simulink model "vel_loop_Bmat"  (Simulink 7.2)
settings: Solver=FixedStepDiscrete  StartTime=0.0  StopTime=0  FixedStep=MACH.dt  RelTol=1e-3
undefined symbols (not defined in the file or in its folder): att_trim_IC, MACH, MACH_mass_IC, MACH_vel_IC, obac_params, u_obac_IC, x_obac_IC
libraries: utility_lib x2, model_lib x2, models x1
settings Model: Creator=E183308  LastModifiedBy=E183308
settings DataIOCC: ExternalInput=[0 d_in]  LoadExternalInput=on  SignalLogging=off  SaveTime=off
settings OptimizationCC: InitFltsAndDblsToZero=on
settings DebuggingCC: SaveWithParameterizedLinksMsg=none  SignalResolutionControl=TryResolveAllWithWarning  InheritedTsInSrcMsg=none  MultiTaskDSMMsg=warning  MultiTaskCondExecSysMsg=none
settings RTWCC: IncludeERTFirstTime=on
settings GRTTargetCC: TargetFcnLib=ansi_tfl_tmw.mat

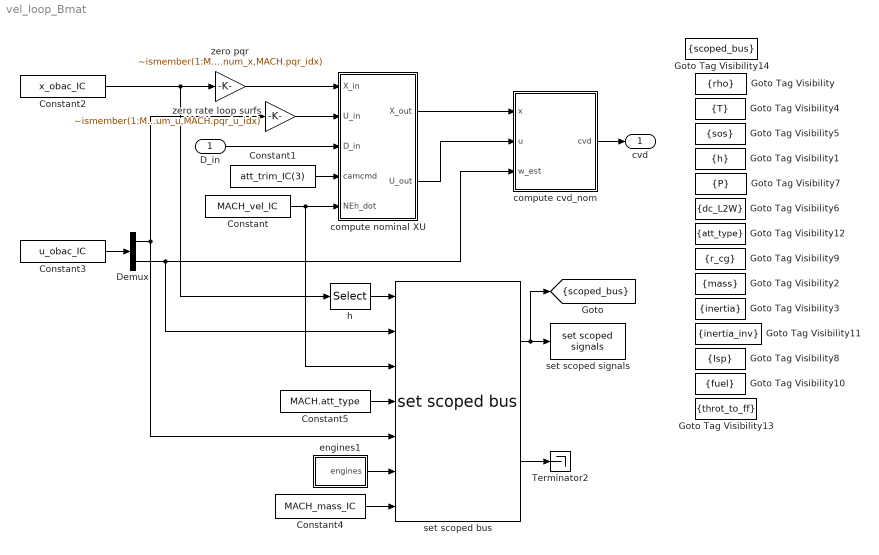
== system vel_loop_Bmat ==
  D_in : Inport  OutDataType=sfix(16)  OutScaling=2^0
  Constant : Constant  Value=MACH_vel_IC  OutDataType=sfix(16)  OutScaling=2^0
  Constant1 : Constant  Value=att_trim_IC(3)  OutDataType=sfix(16)  OutScaling=2^0
  Constant2 : Constant  Value=x_obac_IC  OutDataType=sfix(16)  OutScaling=2^0
  Constant3 : Constant  Value=u_obac_IC  OutDataType=sfix(16)  OutScaling=2^0
  Constant4 : Constant  Value=MACH_mass_IC  OutDataType=sfix(16)  OutScaling=2^0
  Constant5 : Constant  Value=MACH.att_type  OutDataType=sfix(16)  OutScaling=2^0
  Demux : Demux  Outputs=[MACH.num_u 3]
  Goto Tag Visibility : GotoTagVisibility  GotoTag=rho
  Goto Tag Visibility1 : GotoTagVisibility  GotoTag=h
  Goto Tag Visibility10 : GotoTagVisibility  GotoTag=fuel
  Goto Tag Visibility11 : GotoTagVisibility  GotoTag=inertia_inv
  Goto Tag Visibility12 : GotoTagVisibility  GotoTag=att_type
  Goto Tag Visibility13 : GotoTagVisibility  GotoTag=throt_to_ff
  Goto Tag Visibility14 : GotoTagVisibility  GotoTag=scoped_bus
  Goto Tag Visibility2 : GotoTagVisibility  GotoTag=mass
  Goto Tag Visibility3 : GotoTagVisibility  GotoTag=inertia
  Goto Tag Visibility4 : GotoTagVisibility  GotoTag=T
  Goto Tag Visibility5 : GotoTagVisibility  GotoTag=sos
  Goto Tag Visibility6 : GotoTagVisibility  GotoTag=dc_L2W
  Goto Tag Visibility7 : GotoTagVisibility  GotoTag=P
  Goto Tag Visibility8 : GotoTagVisibility  GotoTag=Isp
  Goto Tag Visibility9 : GotoTagVisibility  GotoTag=r_cg
  Terminator2 : Terminator
  compute cvd_nom : Subsystem
  compute nominal XU : Subsystem
  engines1 : Subsystem
  h : Selector  InputPortWidth=obac_params.num_x  IndexOptions=Index vector (dialog)  Indices=MACH.NEh_idx(3)  OutputSizes=1
  set scoped bus : model_lib/set scoped bus  SystemSampleTime=-1  vehicle_params=obac_params
  set scoped signals : model_lib/set scoped signals  SystemSampleTime=-1
  zero pqr : Gain  Gain=~ismember(1:MACH.num_x,MACH.pqr_idx)  ParameterDataType=sfix(16)  ParameterScaling=2^0  OutDataType=sfix(16)  OutScaling=2^0
  zero rate loop surfs : Gain  Gain=~ismember(1:MACH.num_u,MACH.pqr_u_idx)  ParameterDataType=sfix(16)  ParameterScaling=2^0  OutDataType=sfix(16)  OutScaling=2^0
  cvd : Outport  OutDataType=sfix(16)  OutScaling=2^0
  tag scope: scoped_bus=scoped
  wires:
  compute nominal XU/1(X_out) -> compute cvd_nom/1(x)
  Constant/1 -> compute nominal XU/5(NEh_dot), set scoped bus/3
  Constant1/1 -> compute nominal XU/4(camcmd)
  Constant2/1 -> h/1, zero pqr/1
  D_in/1 -> compute nominal XU/3(D_in)
  compute cvd_nom/1(cvd) -> cvd/1
  h/1 -> set scoped bus/1
  Constant5/1 -> set scoped bus/4
  set scoped bus/1 -> set scoped signals/1, [scoped_bus]
  set scoped bus/2 -> Terminator2/1
  compute nominal XU/2(U_out) -> compute cvd_nom/2(u)
  Constant3/1 -> Demux/1
  Demux/2 -> set scoped bus/2, compute cvd_nom/3(w_est)
  Demux/1 -> set scoped bus/5, zero rate loop surfs/1
  zero rate loop surfs/1 -> compute nominal XU/2(U_in)
  zero pqr/1 -> compute nominal XU/1(X_in)
  Constant4/1 -> set scoped bus/7
  engines1/1(engines) -> set scoped bus/6

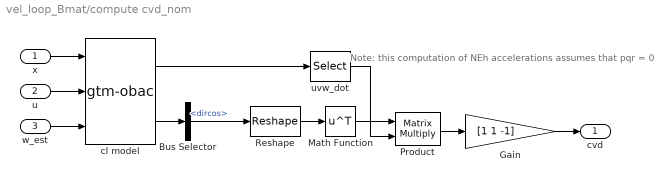
== system vel_loop_Bmat/compute cvd_nom ==
  note: Note: this computation of NEh accelerations
      | assumes that pqr = 0
  x : Inport  OutDataType=sfix(16)  OutScaling=2^0
  u : Inport  Port=2  OutDataType=sfix(16)  OutScaling=2^0
  w_est : Inport  Port=3  OutDataType=sfix(16)  OutScaling=2^0
  Bus Selector : BusSelector  OutputSignals=dircos
  Gain : Gain  Gain=[1 1 -1]  ParameterDataType=sfix(16)  ParameterScaling=2^0  OutDataType=sfix(16)  OutScaling=2^0  SaturateOnIntegerOverflow=on  OutDataTypeStr=Inherit: Same as input  ParamDataTypeStr=Inherit: Same as input
  Math Function : Math  Operator=transpose  OutDataType=sfix(16)  OutScaling=2^0  SaturateOnIntegerOverflow=on
  Product : Product  Multiplication=Matrix(*)  OutDataType=sfix(16)  OutScaling=2^0  SaturateOnIntegerOverflow=on  InputSameDT=on  OutDataTypeStr=Inherit: Same as first input
  Reshape : Reshape  OutputDimensionality=Customize  OutputDimensions=[3,3]
  cl model : models/gtm-obac  SystemSampleTime=-1
  uvw_dot : Selector  InputPortWidth=MACH.num_x  IndexOptions=Index vector (dialog)  Indices=MACH.uvw_idx  OutputSizes=1
  cvd : Outport  OutDataType=sfix(16)  OutScaling=2^0
  wires:
  cl model/2 -> Bus Selector/1
  cl model/1 -> uvw_dot/1
  w_est/1 -> cl model/3
  u/1 -> cl model/2
  Bus Selector/1 -> Reshape/1  "<dircos>"
  Gain/1 -> cvd/1
  Product/1 -> Gain/1
  Math Function/1 -> Product/1
  Reshape/1 -> Math Function/1
  x/1 -> cl model/1
  uvw_dot/1 -> Product/2

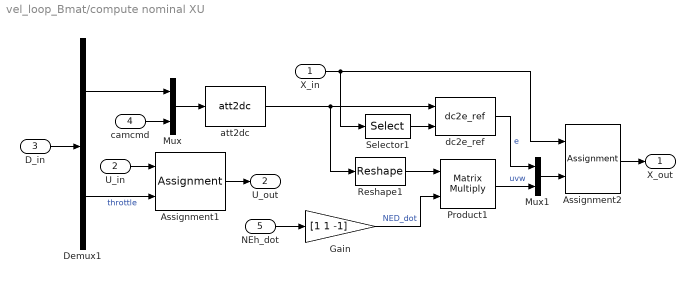
== system vel_loop_Bmat/compute nominal XU ==
  X_in : Inport  OutDataType=sfix(16)  OutScaling=2^0
  U_in : Inport  Port=2  OutDataType=sfix(16)  OutScaling=2^0
  D_in : Inport  Port=3  OutDataType=sfix(16)  OutScaling=2^0
  camcmd : Inport  Port=4  OutDataType=sfix(16)  OutScaling=2^0
  NEh_dot : Inport  Port=5  OutDataType=sfix(16)  OutScaling=2^0
  Assignment1 : Assignment  IndexOptions=Index vector (dialog)  Indices=MACH.throttle_idx  OutputSizes=[1 1]
  Assignment2 : Assignment  IndexOptions=Index vector (dialog)  Indices=[ MACH.quat_idx MACH.uvw_idx]  OutputSizes=[1 1]
  Demux1 : Demux  Outputs=[ 2 length(MACH.throttle_idx) ]
  Gain : Gain  Gain=[1 1 -1]  ParameterDataType=sfix(16)  ParameterScaling=2^0  OutDataType=sfix(16)  OutScaling=2^0  SaturateOnIntegerOverflow=on  OutDataTypeStr=Inherit: Same as input  ParamDataTypeStr=Inherit: Same as input
  Mux : Mux  Inputs=[ 2 1 ]
  Mux1 : Mux  Inputs=2
  Product1 : Product  Multiplication=Matrix(*)  OutDataType=sfix(16)  OutScaling=2^0  SaturateOnIntegerOverflow=on  OutDataTypeStr=Inherit: Same as first input
  Reshape1 : Reshape  OutputDimensionality=Customize  OutputDimensions=[3,3]
  Selector1 : Selector  InputPortWidth=MACH.num_x  IndexOptions=Index vector (dialog)  Indices=MACH.quat_idx  OutputSizes=1
  att2dc : utility_lib/att2dc  SystemSampleTime=-1
  dc2e_ref : utility_lib/dc2e_ref  SystemSampleTime=-1
  X_out : Outport  OutDataType=sfix(16)  OutScaling=2^0
  U_out : Outport  Port=2  OutDataType=sfix(16)  OutScaling=2^0
  wires:
  Mux1/1 -> Assignment2/2
  Product1/1 -> Mux1/2  "uvw"
  Selector1/1 -> dc2e_ref/2
  Gain/1 -> Product1/2  "NED_dot"
  dc2e_ref/1 -> Mux1/1  "e"
  att2dc/1 -> dc2e_ref/1, Reshape1/1
  Assignment2/1 -> X_out/1
  Reshape1/1 -> Product1/1
  NEh_dot/1 -> Gain/1
  Demux1/1 -> Mux/1
  camcmd/1 -> Mux/2
  Assignment1/1 -> U_out/1
  X_in/1 -> Selector1/1, Assignment2/1
  U_in/1 -> Assignment1/1
  D_in/1 -> Demux1/1
  Demux1/2 -> Assignment1/2  "throttle"
  Mux/1 -> att2dc/1

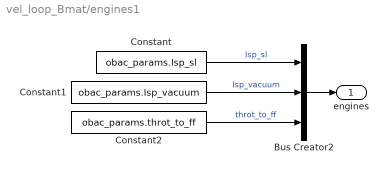
== system vel_loop_Bmat/engines1 ==
  Bus Creator2 : BusCreator  Inputs=3
  Constant : Constant  Value=obac_params.Isp_sl  OutDataType=sfix(16)  OutScaling=2^0
  Constant1 : Constant  Value=obac_params.Isp_vacuum  OutDataType=sfix(16)  OutScaling=2^0
  Constant2 : Constant  Value=obac_params.throt_to_ff  OutDataType=sfix(16)  OutScaling=2^0
  engines : Outport  OutDataType=sfix(16)  OutScaling=2^0
  wires:
  Constant1/1 -> Bus Creator2/2  "Isp_vacuum"
  Constant/1 -> Bus Creator2/1  "Isp_sl"
  Bus Creator2/1 -> engines/1
  Constant2/1 -> Bus Creator2/3  "throt_to_ff"
